simulink model "nsdynamic_Cori_Cent"  (R2021b)
settings: Solver=ode4  StartTime=0.0  StopTime=10.0  RelTol=1e-3
InitFcn:
  | initialization
undefined symbols (not defined in the file or in its folder): dynNS_Cori_Cent, trajectory
settings Model: Creator=AzamaoZ  LastModifiedBy=AzamaoZ

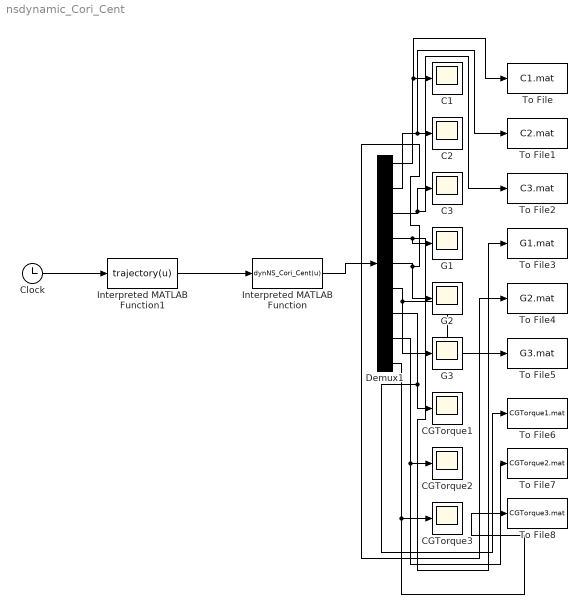
== system nsdynamic_Cori_Cent ==
  C1 : Scope
  C2 : Scope
  C3 : Scope
  CGTorque1 : Scope
  CGTorque2 : Scope
  CGTorque3 : Scope
  Clock : Clock
  Demux1 : Demux  Outputs=9
  G1 : Scope
  G2 : Scope
  G3 : Scope
  Interpreted MATLAB Function : MATLABFcn  MATLABFcn=dynNS_Cori_Cent(u)  OutputDimensions=9
  Interpreted MATLAB Function1 : MATLABFcn  MATLABFcn=trajectory(u)
  To File : ToFile  Filename=C1.mat  MatrixName=C1  SaveFormat=Timeseries
  To File1 : ToFile  Filename=C2.mat  MatrixName=C2  SaveFormat=Timeseries
  To File2 : ToFile  Filename=C3.mat  MatrixName=C3  SaveFormat=Timeseries
  To File3 : ToFile  Filename=G1.mat  MatrixName=G1  SaveFormat=Timeseries
  To File4 : ToFile  Filename=G2.mat  MatrixName=G2  SaveFormat=Timeseries
  To File5 : ToFile  Filename=G3.mat  MatrixName=G3  SaveFormat=Timeseries
  To File6 : ToFile  Filename=CGTorque1.mat  MatrixName=CGTorque1  SaveFormat=Timeseries
  To File7 : ToFile  Filename=CGTorque2.mat  MatrixName=CGTorque2  SaveFormat=Timeseries
  To File8 : ToFile  Filename=CGTorque3.mat  MatrixName=CGTorque3  SaveFormat=Timeseries
  wires:
  Interpreted MATLAB Function/1 -> Demux1/1
  Clock/1 -> Interpreted MATLAB Function1/1
  Demux1/1 -> To File/1, C1/1
  Demux1/8 -> To File7/1, CGTorque2/1
  Demux1/2 -> To File1/1, C2/1
  Demux1/7 -> To File6/1, CGTorque1/1
  Demux1/9 -> To File8/1, CGTorque3/1
  Demux1/4 -> To File3/1, G1/1
  Demux1/6 -> To File5/1, G3/1
  Demux1/5 -> To File4/1, G2/1
  Demux1/3 -> To File2/1, C3/1
  Interpreted MATLAB Function1/1 -> Interpreted MATLAB Function/1
